simulink model "Flightinstrument"  (R2021b)
settings: Solver=VariableStepAuto  StartTime=0.0  StopTime=10.0  RelTol=1e-3
PreLoadFcn:
  | % Bus object: States
  | clear templateElems;
  | templateElems(1) = Simulink.BusElement;
  | templateElems(1).Name = 'V_body';
  | templateElems(1).Dimensions = [3 1];
  | templateElems(1).DimensionsMode = 'Fixed';
  | templateElems(1).DataType = 'double';
  | templateElems(1).SampleTime = -1;
  | templateElems(1).Complexity = 'real';
  | templateElems(1).SamplingMode = 'Sample based';
  | templateElems(1).Min = [];
  | templateElems(1).Max = [];
  | templateElems(1).DocUnits = '';
  | templateElems(1).Description = '';
  | 
  | templateElems(2) = Simulink.BusElement;
  | templateElems(2).Name = 'Omega_body';
  | templateElems(2).Dimensions = [3 1];
  | templateElems(2).DimensionsMode = 'Fixed';
  | templateElems(2).DataType = 'double';
  | templateElems(2).SampleTime = -1;
  | templateElems(2).Complexity = 'real';
  | templateElems(2).SamplingMode = 'Sample based';
  | templateElems(2).Min = [];
  | templateElems(2).Max = [];
  | templateElems(2).DocUnits = '';
  | templateElems(2).Description = '';
  | 
  | templateElems(3) = Simulink.BusElement;
  | templateElems(3).Name = 'Euler';
  | templateElems(3).Dimensions = [3 1];
  | templateElems(3).DimensionsMode = 'Fixed';
  | templateElems(3).DataType = 'double';
  | templateElems(3).SampleTime = -1;
  | templateElems(3).Complexity = 'real';
  | templateElems(3).SamplingMode = 'Sample based';
  | templateElems(3).Min = [];
  | templateElems(3).Max = [];
  | templateElems(3).DocUnits = '';
  | templateElems(3).Description = '';
  | 
  | templateElems(4) = Simulink.BusElement;
  | templateElems(4).Name = 'Accel_body';
  | templateElems(4).Dimensions = [3 1];
  | templateElems(4).DimensionsMode = 'Fixed';
  | templateElems(4).DataType = 'double';
  | templateElems(4).SampleTime = -1;
  | templateElems(4).Complexity = 'real';
  | templateElems(4).SamplingMode = 'Sample based';
  | templateElems(4).Min = [];
  | templateElems(4).Max = [];
  | templateElems(4).DocUnits = '';
  | templateElems(4).Description = '';
  | 
  | templateElems(5) = Simulink.BusElement;
  | templateElems(5).Name = 'dOmega_body';
  | templateElems(5).Dimensions = [3 1];
  | templateElems(5).DimensionsMode = 'Fixed';
  | templateElems(5).DataType = 'double';
  | templateElems(5).SampleTime = -1;
  | templateElems(5).Complexity = 'real';
  | templateElems(5).SamplingMode = 'Sample based';
  | templateElems(5).Min = [];
  | templateElems(5).Max = [];
  | templateElems(5).DocUnits = '';
  | templateElems(5).Description = '';
  | 
  | templateElems(6) = Simulink.BusElement;
  | templateElems(6).Name = 'V_ned';
  | templateElems(6).Dimensions = [3 1];
  | templateElems(6).DimensionsMode = 'Fixed';
  | templateElems(6).DataType = 'double';
  | templateElems(6).SampleTime = -1;
  | templateElems(6).Complexity = 'real';
  | templateElems(6).SamplingMode = 'Sample based';
  | templateElems(6).Min = [];
  | templateElems(6).Max = [];
  | templateElems(6).DocUnits = '';
  | templateElems(6).Description = '';
  | 
  | templateElems(7) = Simulink.BusElement;
  | templateElems(7).Name = 'X_ned';
  | templateElems(7).Dimensions = [3 1];
  | templateElems(7).DimensionsMode = 'Fixed';
  | templateElems(7).DataType = 'double';
  | templateElems(7).SampleTime = -1;
  | templateElems(7).Complexity = 'real';
  | templateElems(7).SamplingMode = 'Sample based';
  | templateElems(7).Min = [];
  | templateElems(7).Max = [];
  | templateElems(7).DocUnits = '';
  | templateElems(7).Description = '';
  | 
  | templateElems(8) = Simulink.BusElement;
  | templateElems(8).Name = 'LLA';
  | templateElems(8).Dimensions = [1 3];
  | templateElems(8).DimensionsMode = 'Fixed';
  | templateElems(8).DataType = 'double';
  | templateElems(8).SampleTime = -1;
  | templateElems(8).Complexity = 'real';
  | templateElems(8).SamplingMode = 'Sample based';
  | templateElems(8).Min = [];
  | templateElems(8).Max = [];
  | templateElems(8).DocUnits = '';
  | templateElems(8).Description = sprintf('Latitude, Longitude, Altitude');
  | 
  | templateElems(9) = Simulink.BusElement;
  | templateElems(9).Name = 'DCM_be';
  | templateElems(9).Dimensions = [3 3];
  | templateElems(9).DimensionsMode = 'Fixed';
  | templateElems(9).DataType = 'double';
  | templateElems(9).SampleTime = -1;
  | templateElems(9).Complexity = 'real';
  | templateElems(9).SamplingMode = 'Sample based';
  | templateElems(9).Min = [];
  | templateElems(9).Max = [];
  | templateElems(9).DocUnits = '';
  | templateElems(9).Description = '';
  | 
  | 
  | AirframeStatesBus = Simulink.Bus;
  | AirframeStatesBus.HeaderFile = '';
  | AirframeStatesBus.Description = '';
  | AirframeStatesBus.DataScope = 'Auto';
  | AirframeStatesBus.Alignment = -1;
  | AirframeStatesBus.Elements = templateElems;
  | clear templateElems;
undefined symbols (not defined in the file or in its folder): deg, Earth, ft, m, rad, s, WGS84
libraries: aerolibconvert2 x7, aerolibasang x3, shared6dof x1, aerolibadyn x1, aerolibactuator x1, aerolibtransform2 x1, aerolibnav x1
settings Model: Creator=asus  LastModifiedBy=asus
settings SolverCC: AlgebraicLoopSolver=TrustRegion  MinimalZcImpactIntegration=on
settings DebuggingCC: PregeneratedLibrarySubsystemCodeDiagnostic=none  SFMachineParentedDataDiag=warning  ArithmeticOperatorsInVariantConditions=warning
settings SFSimCC: SimUseLocalCustomCode=off
settings RTWCC: RTWUseLocalCustomCode=off

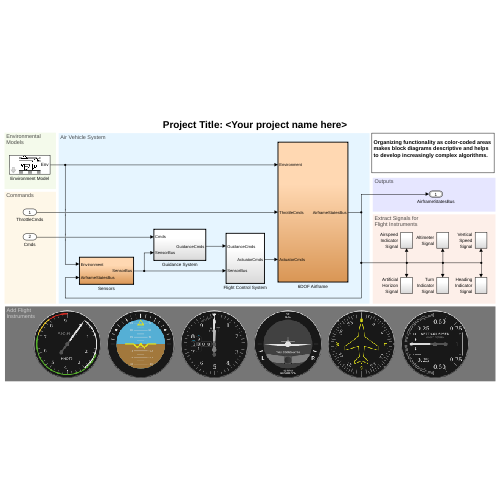
[thumbnail: Simulink's stored preview of the top-level diagram]
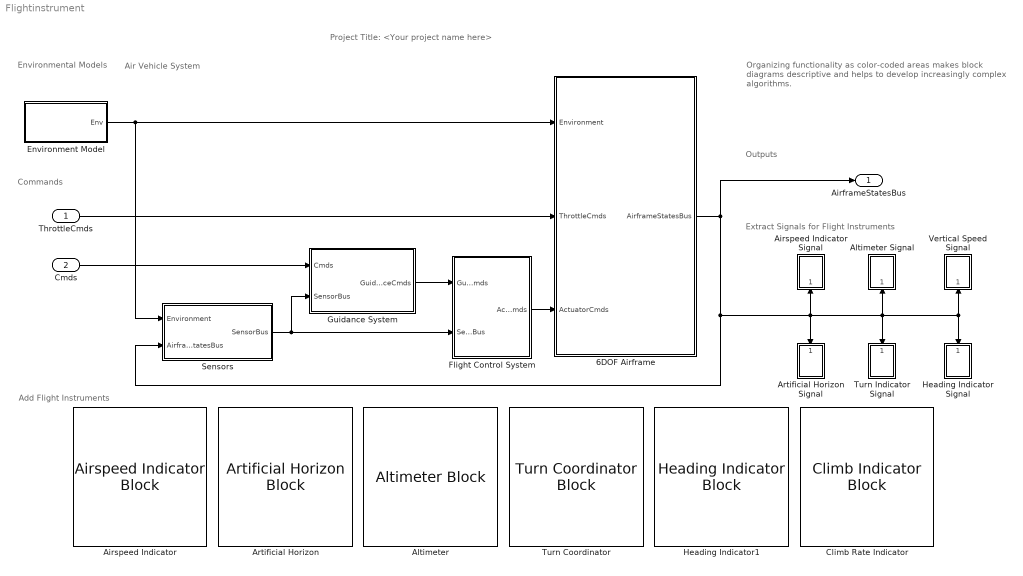
== system Flightinstrument ==
  note: Organizing functionality as color-coded areas makes block diagrams descriptive and helps to develop increasingly complex algorithms.
  note: Project Title: <Your project name here>
  note: Air Vehicle System
  note: Extract Signals for
      | Flight Instruments
  note: Add Flight
      | Instruments
  note: Outputs
  note: Environmental
      | Models
  note: Commands
  ThrottleCmds : Inport
  Cmds : Inport  Port=2
  6DOF Airframe : Subsystem  TreatAsAtomicUnit=on
  Airspeed Indicator Signal : Subsystem
  Airspeed Indicator : AirspeedIndicatorBlock  LabelPosition=Hide  ScaleMin=0  ScaleMax=9
  Altimeter : AltimeterBlock  LabelPosition=Hide
  Altimeter Signal : Subsystem
  Artificial Horizon Signal : Subsystem
  Artificial Horizon : ArtificialHorizonBlock  LabelPosition=Hide
  Climb Rate Indicator : ClimbIndicatorBlock  LabelPosition=Hide  ScaleMax=1000
  Environment Model : Subsystem  mask(Constant Environment Model){To=288, a=340, Po=101.3e3, AirDensity=1.229, ugvgwg=[0 0 0], pgqgrg=[0 0 0], g=[0 0 9.81]}
      mask prompts: To "Constant Temperature (K):"; a "Constant Speed of Sound (m/s):"; Po "Constant Pressure (Pa):"; AirDensity "Constant Air Density (kg/m^3):"; ugvgwg "Constant Wind Velocity [ug vg wg] (m/s):"; pgqgrg "Constant Wind Angular Rates [pg qg rg] (rad/s):"; g "Constant Gravitational Acceleration (m/s^2):"
      mask Help: helpview(fullfile(docroot,'toolbox','aeroblks','aeroblks.map'), 'environment1');
      mask TypeOptions To: Constant Atmosphere/To
      mask TypeOptions a: Constant Atmosphere/a
      mask TypeOptions Po: Constant Atmosphere/Po
      mask TypeOptions AirDensity: Constant Atmosphere/AirDensity
      mask TypeOptions ugvgwg: Constant Wind/ugvgwg
      mask TypeOptions pgqgrg: Constant Wind/pgqgrg
      mask TypeOptions g: Constant Gravity/g
      mask DialogControl Container4 Prompt: Atmospheric Model
      mask DialogControl Container6 Prompt: Wind Model
      mask DialogControl Container8 Prompt: Gravity Model
      mask Display:
      | image('aeroenvironment.bmp','center')
      | port_label('output',1,'Env')
  Flight Control System : Subsystem  TreatAsAtomicUnit=on
  Guidance System : Subsystem  TreatAsAtomicUnit=on
  Heading Indicator Signal : Subsystem
  Heading Indicator1 : HeadingIndicatorBlock  LabelPosition=Hide
  Sensors : Subsystem  TreatAsAtomicUnit=on  VariantControl=VSS_SENSORS_DYNAMICS
  Turn Indicator Signal : Subsystem
  Turn Coordinator : TurnCoordinatorBlock  LabelPosition=Hide
  Vertical Speed Signal : Subsystem
  AirframeStatesBus : Outport  OutDataTypeStr=Bus: AirframeStatesBus  VectorParamsAs1DForOutWhenUnconnected=off
  wires:
  6DOF Airframe/1(AirframeStatesBus) -> Sensors/2(AirframeStatesBus), Altimeter Signal/1(AirframeStatesBus), Heading Indicator Signal/1(AirframeStatesBus), Vertical Speed Signal/1(AirframeStatesBus), Turn Indicator Signal/1(AirframeStatesBus), Airspeed Indicator Signal/1(AirframeStatesBus), Artificial Horizon Signal/1(AirframeStatesBus), AirframeStatesBus/1
  Cmds/1 -> Guidance System/1(Cmds)
  Guidance System/1(GuidanceCmds) -> Flight Control System/1(GuidanceCmds)
  Sensors/1(SensorBus) -> Guidance System/2(SensorBus), Flight Control System/2(SensorBus)
  ThrottleCmds/1 -> 6DOF Airframe/2(ThrottleCmds)
  Environment Model/1(Env) -> Sensors/1(Environment), 6DOF Airframe/1(Environment)
  Flight Control System/1(ActuatorCmds) -> 6DOF Airframe/3(ActuatorCmds)

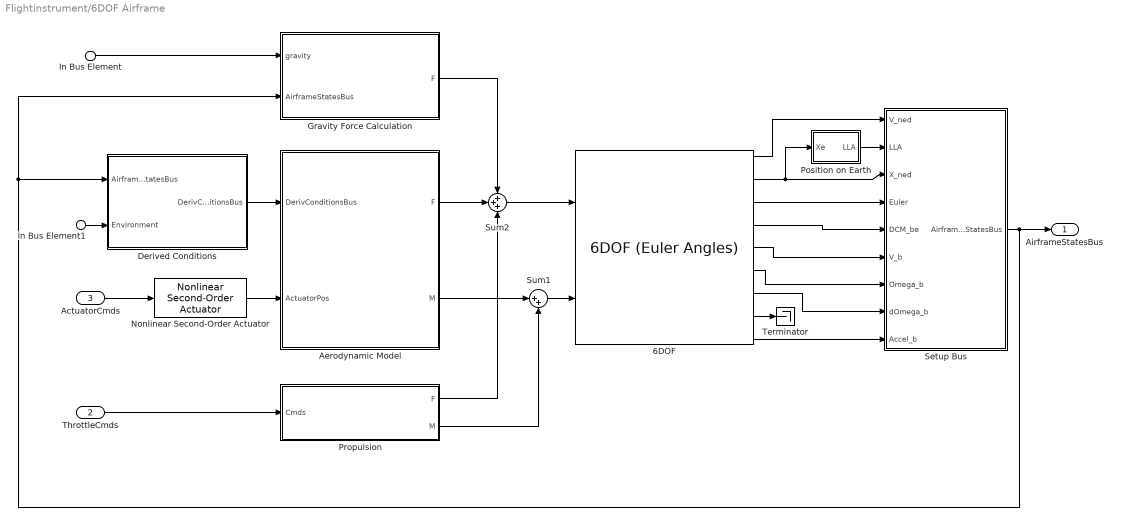
== system Flightinstrument/6DOF Airframe ==
  In Bus Element1 : Inport  PortName=Environment
  In Bus Element : Inport  PortName=Environment  Element=g
  ThrottleCmds : Inport  Port=2
  ActuatorCmds : Inport  Port=3
  6DOF : shared6dof/6DOF (Euler Angles)  units=Metric (MKS)  mtype=Fixed  rep=Euler Angles  xme_0=[0 0 -1000]  Vm_0=[100 0 0]  eul_0=[0 0 0]  pm_0=[0 0 0]  mass_0=1000  mass_e=0.5  mass_f=2.0  inertia=eye(3)  inertia_e=eye(3)  inertia_f=2*eye(3)  k_quat=Vehicle.SixDOF.quatGain  vre_flag=on  abi_flag=on  aMode=0  xme_statename=''  Vm_statename=''  eul_statename=''  quat_statename=''  pm_statename=''  mass_statename=''
      settings: SourceProductBaseCode=AE,PW,DR,MT,UV,VE
  Aerodynamic Model : Subsystem
  Derived Conditions : Subsystem
  Gravity Force Calculation : Subsystem
  Nonlinear Second-Order Actuator : aerolibactuator/Nonlinear Second-Order Actuator  wn_fin=1  z_fin=0.3  fin_max=20*pi/180  fin_min=-20*pi/180  fin_maxrate=500*pi/180  fin_act_0=0  fin_act_vel=0
      settings: SourceProductBaseCode=AE
  Position on Earth : Subsystem  Priority=1  TreatAsAtomicUnit=on
  Propulsion : Subsystem
  Setup Bus : Subsystem
  Sum1 : Sum  Inputs=|++  InputSameDT=on  SaturateOnIntegerOverflow=on  OutDataTypeStr=Inherit: Same as first input
  Sum2 : Sum  Inputs=+++  InputSameDT=on  SaturateOnIntegerOverflow=on  OutDataTypeStr=Inherit: Same as first input
  Terminator : Terminator
  AirframeStatesBus : Outport  OutDataTypeStr=Bus: AirframeStatesBus  VectorParamsAs1DForOutWhenUnconnected=off
  wires:
  Setup Bus/1(AirframeStatesBus) -> AirframeStatesBus/1, Gravity Force Calculation/2(AirframeStatesBus), Derived Conditions/1(AirframeStatesBus)
  6DOF/1 -> Setup Bus/1(V_ned)
  Derived Conditions/1(DerivConditionsBus) -> Aerodynamic Model/1(DerivConditionsBus)
  In Bus Element1/1 -> Derived Conditions/2(Environment)
  Aerodynamic Model/2(M) -> Sum1/1
  ThrottleCmds/1 -> Propulsion/1(Cmds)
  ActuatorCmds/1 -> Nonlinear Second-Order Actuator/1
  Nonlinear Second-Order Actuator/1 -> Aerodynamic Model/2(ActuatorPos)
  Propulsion/1(F) -> Sum2/3
  Propulsion/2(M) -> Sum1/2
  6DOF/5 -> Setup Bus/6(V_b)
  Aerodynamic Model/1(F) -> Sum2/2
  6DOF/4 -> Setup Bus/5(DCM_be)
  Gravity Force Calculation/1(F) -> Sum2/1
  In Bus Element/1 -> Gravity Force Calculation/1(gravity)
  6DOF/9 -> Setup Bus/9(Accel_b)
  Sum2/1 -> 6DOF/1
  Sum1/1 -> 6DOF/2
  6DOF/2 -> Position on Earth/1(Xe), Setup Bus/3(X_ned)
  6DOF/3 -> Setup Bus/4(Euler)
  6DOF/6 -> Setup Bus/7(Omega_b)
  6DOF/7 -> Setup Bus/8(dOmega_b)
  Position on Earth/1(LLA) -> Setup Bus/2(LLA)
  6DOF/8 -> Terminator/1

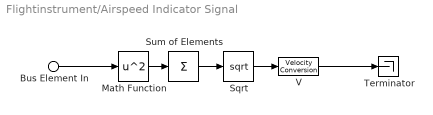
== system Flightinstrument/Airspeed Indicator Signal ==
  Bus Element In : Inport  PortName=AirframeStatesBus  Element=V_body
  Math Function : Math  Operator=square  SignedPower=on  SaturateOnIntegerOverflow=on
  Sqrt : Sqrt  SaturateOnIntegerOverflow=on
  Sum of Elements : Sum  Inputs=+
  Terminator : Terminator
  V : aerolibconvert2/Velocity Conversion  IU=m/s  OU=kts
  wires:
  Bus Element In/1 -> Math Function/1
  V/1 -> Terminator/1
  Sqrt/1 -> V/1
  Math Function/1 -> Sum of Elements/1
  Sum of Elements/1 -> Sqrt/1

== system Flightinstrument/Altimeter Signal ==
  Bus Element In : Inport  PortName=AirframeStatesBus  Element=LLA
  Altitude [ft] : aerolibconvert2/Length Conversion  IU=m  OU=ft
  Altitude [m] : Selector  InputPortWidth=3  IndexOptions=Index vector (dialog)  Indices=[3]  OutputSizes=1
  Terminator : Terminator
  wires:
  Bus Element In/1 -> Altitude [m]/1
  Altitude [ft]/1 -> Terminator/1
  Altitude [m]/1 -> Altitude [ft]/1

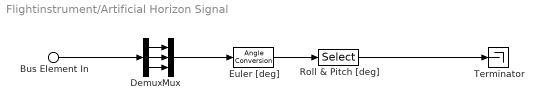
== system Flightinstrument/Artificial Horizon Signal ==
  Bus Element In : Inport  PortName=AirframeStatesBus  Element=Euler
  Demux : Demux  Outputs=3
  Euler [deg] : aerolibconvert2/Angle Conversion  IU=rad  OU=deg
  Mux : Mux  Inputs=3
  Roll & Pitch [deg] : Selector  InputPortWidth=3  IndexOptions=Index vector (dialog)  Indices=[1 2]  OutputSizes=1
  Terminator : Terminator
  wires:
  Roll & Pitch [deg]/1 -> Terminator/1
  Mux/1 -> Euler [deg]/1
  Demux/3 -> Mux/3
  Demux/1 -> Mux/1
  Demux/2 -> Mux/2
  Bus Element In/1 -> Demux/1
  Euler [deg]/1 -> Roll & Pitch [deg]/1

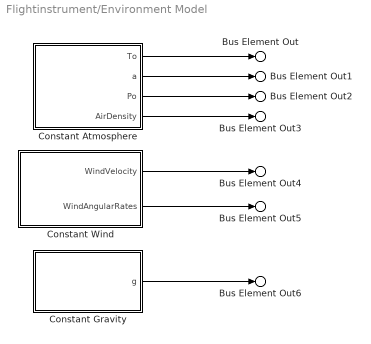
== system Flightinstrument/Environment Model ==
  Constant Atmosphere : Subsystem  VariantControl=atmosCONST  mask(Standard Atmospheric Constants){To=To, a=a, Po=Po, AirDensity=AirDensity}
      mask prompts: To "Constant Temperature (K):"; a "Constant Speed of Sound (m/s):"; Po "Constant Pressure (Pa):"; AirDensity "Constant Air Density (kg/m^3):"
  Constant Gravity : Subsystem  VariantControl=gravCONST  mask(Constant Gravitational Acceleration){g=g}
      mask prompts: g "Constant Gravitational Acceleration (m/s^2):"
  Constant Wind : Subsystem  VariantControl=windCONST  mask(Constant Wind Values){ugvgwg=ugvgwg, pgqgrg=pgqgrg}
      mask prompts: ugvgwg "Constant Wind Velocity (m/s):"; pgqgrg "Constant Wind Angular Rates (rad/s):"
  Bus Element Out : Outport  VectorParamsAs1DForOutWhenUnconnected=off  PortName=Env  Element=To
  Bus Element Out1 : Outport  VectorParamsAs1DForOutWhenUnconnected=off  PortName=Env  Element=a
  Bus Element Out2 : Outport  VectorParamsAs1DForOutWhenUnconnected=off  PortName=Env  Element=Po
  Bus Element Out3 : Outport  VectorParamsAs1DForOutWhenUnconnected=off  PortName=Env  Element=AirDensity
  Bus Element Out4 : Outport  VectorParamsAs1DForOutWhenUnconnected=off  PortName=Env  Element=WindVelocity
  Bus Element Out5 : Outport  VectorParamsAs1DForOutWhenUnconnected=off  PortName=Env  Element=WindAngularRates
  Bus Element Out6 : Outport  VectorParamsAs1DForOutWhenUnconnected=off  PortName=Env  Element=g
  wires:
  Constant Wind/2(WindAngularRates) -> Bus Element Out5/1
  Constant Atmosphere/3(Po) -> Bus Element Out2/1
  Constant Atmosphere/4(AirDensity) -> Bus Element Out3/1
  Constant Atmosphere/1(To) -> Bus Element Out/1
  Constant Wind/1(WindVelocity) -> Bus Element Out4/1
  Constant Atmosphere/2(a) -> Bus Element Out1/1
  Constant Gravity/1(g) -> Bus Element Out6/1

== system Flightinstrument/Flight Control System ==
  note: Add Flight Control System Algorithms
  GuidanceCmds : Inport
  SensorBus : Inport  Port=2
  Bus to Vector : BusToVector
  Terminator1 : Terminator
  ActuatorCmds : Outport  VectorParamsAs1DForOutWhenUnconnected=off
  wires:
  GuidanceCmds/1 -> Bus to Vector/1
  Bus to Vector/1 -> ActuatorCmds/1
  SensorBus/1 -> Terminator1/1

== system Flightinstrument/Guidance System ==
  note: Add Guidance System Algorithms
  Cmds : Inport
  SensorBus : Inport  Port=2
  Ground : Ground
  Terminator1 : Terminator
  Terminator2 : Terminator
  GuidanceCmds : Outport  VectorParamsAs1DForOutWhenUnconnected=off
  wires:
  Cmds/1 -> Terminator2/1
  Ground/1 -> GuidanceCmds/1
  SensorBus/1 -> Terminator1/1

== system Flightinstrument/Heading Indicator Signal ==
  note: Customize Deg from North per simulation
  Bus Element In : Inport  PortName=AirframeStatesBus  Element=Euler
  Deg from North : Bias
  Euler [deg] : aerolibconvert2/Angle Conversion  IU=rad  OU=deg
  Terminator : Terminator
  Yaw [deg] : Selector  InputPortWidth=3  IndexOptions=Index vector (dialog)  Indices=[3]  OutputSizes=1
  wires:
  Euler [deg]/1 -> Yaw [deg]/1
  Deg from North/1 -> Terminator/1
  Yaw [deg]/1 -> Deg from North/1
  Bus Element In/1 -> Euler [deg]/1

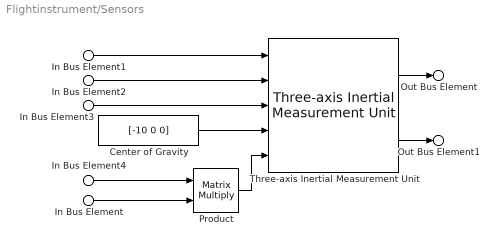
== system Flightinstrument/Sensors ==
  In Bus Element : Inport  PortName=Environment  Element=g
  In Bus Element1 : Inport  Port=2  PortName=AirframeStatesBus  Element=Accel_body
  In Bus Element2 : Inport  Port=2  PortName=AirframeStatesBus  Element=Omega_body
  In Bus Element3 : Inport  Port=2  PortName=AirframeStatesBus  Element=dOmega_body
  In Bus Element4 : Inport  Port=2  PortName=AirframeStatesBus  Element=DCM_be
  Center of Gravity : Constant  Value=[-10 0 0]
  Product : Product  Multiplication=Matrix(*)
  Three-axis Inertial Measurement Unit : aerolibnav/Three-axis Inertial Measurement Unit  units=Metric (MKS)  imu=[0 0 0]  i_Ts=0  dtype_a=on  w_a=190  z_a=0.707  a_sf_cc=[1 0 0; 0 1 0; 0 0 1]  a_bias=[0 0 0]  a_sat="[-inf  -inf  -inf  inf inf inf]"  dtype_g=on  w_g=190  z_g=0.707  g_sf_cc=[1 0 0; 0 1 0; 0 0 1]  g_bias=[0 0 0]  g_sens=[0 0 0]  g_sat="[-inf  -inf  -inf  inf inf inf]"  i_rand=on  i_seeds=[23093 23094 23095 23096 23097 23098]  i_pow=[0.001 0.001 0.001 0.0001 0.0001 0.0001]
  Out Bus Element : Outport  VectorParamsAs1DForOutWhenUnconnected=off  PortName=SensorBus  Element=Accel_body_meas
  Out Bus Element1 : Outport  VectorParamsAs1DForOutWhenUnconnected=off  PortName=SensorBus  Element=Omega_body_meas
  wires:
  In Bus Element/1 -> Product/2
  In Bus Element4/1 -> Product/1
  Three-axis Inertial Measurement Unit/2 -> Out Bus Element1/1
  Three-axis Inertial Measurement Unit/1 -> Out Bus Element/1
  Product/1 -> Three-axis Inertial Measurement Unit/5
  Center of Gravity/1 -> Three-axis Inertial Measurement Unit/4
  In Bus Element3/1 -> Three-axis Inertial Measurement Unit/3
  In Bus Element2/1 -> Three-axis Inertial Measurement Unit/2
  In Bus Element1/1 -> Three-axis Inertial Measurement Unit/1

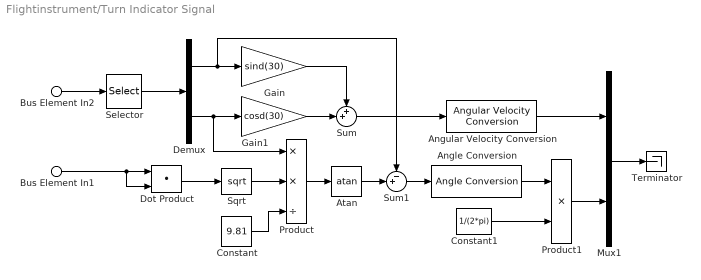
== system Flightinstrument/Turn Indicator Signal ==
  Bus Element In1 : Inport  PortName=AirframeStatesBus  Element=V_body
  Bus Element In2 : Inport  PortName=AirframeStatesBus  Element=Omega_body
  Angle Conversion : aerolibconvert2/Angle Conversion  IU=rad  OU=deg
  Angular Velocity Conversion : aerolibconvert2/Angular Velocity Conversion  IU=rad/s  OU=deg/s
  Atan : Trigonometry  Operator=atan
  Constant : Constant  Value=9.81
  Constant1 : Constant  Value=1/(2*pi)
  Demux : Demux  Outputs=2
  Dot Product : DotProduct  InputSameDT=on  OutDataTypeStr=Inherit: Inherit via internal rule
  Gain : Gain  Gain=sind(30)
  Gain1 : Gain  Gain=cosd(30)
  Mux1 : Mux  Inputs=2
  Product : Product  Inputs=**/
  Product1 : Product  Inputs=**
  Selector : Selector  InputPortWidth=3  IndexOptions=Index vector (dialog)  Indices=[1 3]  OutputSizes=1
  Sqrt : Sqrt  SaturateOnIntegerOverflow=on
  Sum : Sum  Inputs=++|
  Sum1 : Sum  Inputs=-+|
  Terminator : Terminator
  wires:
  Product1/1 -> Mux1/2
  Constant1/1 -> Product1/2
  Sum1/1 -> Angle Conversion/1
  Atan/1 -> Sum1/2
  Constant/1 -> Product/3
  Product/1 -> Atan/1
  Sqrt/1 -> Product/2
  Bus Element In1/1 -> Dot Product/1, Dot Product/2
  Dot Product/1 -> Sqrt/1
  Sum/1 -> Angular Velocity Conversion/1
  Gain1/1 -> Sum/2
  Gain/1 -> Sum/1
  Demux/2 -> Gain1/1, Product/1
  Demux/1 -> Sum1/1, Gain/1
  Selector/1 -> Demux/1
  Bus Element In2/1 -> Selector/1
  Angular Velocity Conversion/1 -> Mux1/1
  Angle Conversion/1 -> Product1/1
  Mux1/1 -> Terminator/1

== system Flightinstrument/Vertical Speed Signal ==
  Bus Element In : Inport  PortName=AirframeStatesBus  Element=V_ned
  Gain : Gain  Gain=-1/1000
  Terminator : Terminator
  Vd [ft/min] : aerolibconvert2/Velocity Conversion  IU=m/s  OU=ft/min
  Vd [m/s] : Selector  InputPortWidth=3  IndexOptions=Index vector (dialog)  Indices=[3]  OutputSizes=1
  wires:
  Gain/1 -> Terminator/1
  Bus Element In/1 -> Vd [m/s]/1
  Vd [m/s]/1 -> Vd [ft/min]/1
  Vd [ft/min]/1 -> Gain/1

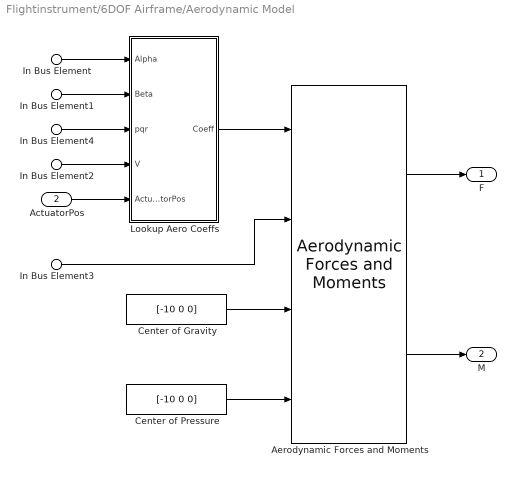
== system Flightinstrument/6DOF Airframe/Aerodynamic Model ==
  In Bus Element : Inport  PortName=DerivConditionsBus  Element=Alpha
  In Bus Element1 : Inport  PortName=DerivConditionsBus  Element=Beta
  In Bus Element2 : Inport  PortName=DerivConditionsBus  Element=Airspeed
  In Bus Element3 : Inport  PortName=DerivConditionsBus  Element=qbar
  In Bus Element4 : Inport  PortName=DerivConditionsBus  Element=Omega_total
  ActuatorPos : Inport  Port=2
  "Aerodynamic Forces and Moments " : aerolibadyn/Aerodynamic Forces and Moments   inputAxes=Body  outputForceAxes=Body  outputMomentAxes=Body  S=1  b=1  cbar=1
  Center of Gravity : Constant  Value=[-10 0 0]
  Center of Pressure : Constant  Value=[-10 0 0]
  Lookup Aero Coeffs : Subsystem
  F : Outport  Unit=N  VectorParamsAs1DForOutWhenUnconnected=off
  M : Outport  Port=2  Unit=N  VectorParamsAs1DForOutWhenUnconnected=off
  wires:
  In Bus Element4/1 -> Lookup Aero Coeffs/3(pqr)
  In Bus Element3/1 -> "Aerodynamic Forces and Moments "/2
  In Bus Element2/1 -> Lookup Aero Coeffs/4(V)
  In Bus Element1/1 -> Lookup Aero Coeffs/2(Beta)
  Center of Pressure/1 -> "Aerodynamic Forces and Moments "/4
  Center of Gravity/1 -> "Aerodynamic Forces and Moments "/3
  ActuatorPos/1 -> Lookup Aero Coeffs/5(ActuatorPos)
  Lookup Aero Coeffs/1(Coeff) -> "Aerodynamic Forces and Moments "/1
  "Aerodynamic Forces and Moments "/1 -> F/1
  "Aerodynamic Forces and Moments "/2 -> M/1
  In Bus Element/1 -> Lookup Aero Coeffs/1(Alpha)

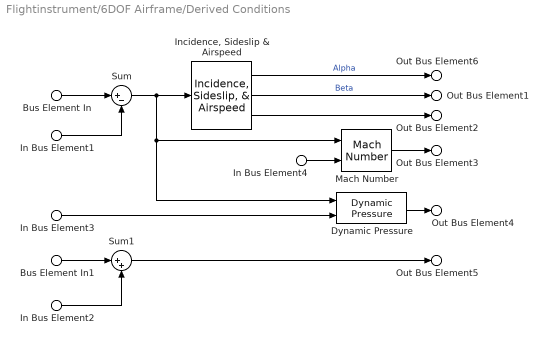
== system Flightinstrument/6DOF Airframe/Derived Conditions ==
  Bus Element In : Inport  PortName=AirframeStatesBus  Element=V_body
  Bus Element In1 : Inport  PortName=AirframeStatesBus  Element=Omega_body
  In Bus Element1 : Inport  Port=2  PortName=Environment  Element=WindVelocity
  In Bus Element2 : Inport  Port=2  PortName=Environment  Element=WindAngularRates
  In Bus Element3 : Inport  Port=2  PortName=Environment  Element=AirDensity
  In Bus Element4 : Inport  Port=2  PortName=Environment  Element=a
  Dynamic Pressure : aerolibasang/Dynamic Pressure
  "Incidence, Sideslip & Airspeed" : aerolibasang/Incidence, Sideslip, & Airspeed
  Mach Number : aerolibasang/Mach Number
      settings: SourceProductBaseCode=AE
  Sum : Sum  Inputs=|+-  InputSameDT=on  SaturateOnIntegerOverflow=on  OutDataTypeStr=Inherit: Same as first input
  Sum1 : Sum  Inputs=|++  InputSameDT=on  SaturateOnIntegerOverflow=on  OutDataTypeStr=Inherit: Same as first input
  Out Bus Element6 : Outport  VectorParamsAs1DForOutWhenUnconnected=off  PortName=DerivConditionsBus  Element=Alpha
  Out Bus Element1 : Outport  VectorParamsAs1DForOutWhenUnconnected=off  PortName=DerivConditionsBus  Element=Beta
  Out Bus Element2 : Outport  VectorParamsAs1DForOutWhenUnconnected=off  PortName=DerivConditionsBus  Element=Airspeed
  Out Bus Element3 : Outport  VectorParamsAs1DForOutWhenUnconnected=off  PortName=DerivConditionsBus  Element=Mach
  Out Bus Element4 : Outport  VectorParamsAs1DForOutWhenUnconnected=off  PortName=DerivConditionsBus  Element=qbar
  Out Bus Element5 : Outport  VectorParamsAs1DForOutWhenUnconnected=off  PortName=DerivConditionsBus  Element=Omega_total
  wires:
  In Bus Element1/1 -> Sum/2
  In Bus Element2/1 -> Sum1/2
  Sum1/1 -> Out Bus Element5/1
  Bus Element In1/1 -> Sum1/1
  "Incidence, Sideslip & Airspeed"/1 -> Out Bus Element6/1  "Alpha"
  "Incidence, Sideslip & Airspeed"/2 -> Out Bus Element1/1  "Beta"
  In Bus Element4/1 -> Mach Number/2
  Bus Element In/1 -> Sum/1
  Sum/1 -> "Incidence, Sideslip & Airspeed"/1, Mach Number/1, Dynamic Pressure/1
  Mach Number/1 -> Out Bus Element3/1
  In Bus Element3/1 -> Dynamic Pressure/2
  Dynamic Pressure/1 -> Out Bus Element4/1
  "Incidence, Sideslip & Airspeed"/3 -> Out Bus Element2/1

== system Flightinstrument/6DOF Airframe/Gravity Force Calculation ==
  gravity : Inport  Unit=m/s^2
  Bus Element In : Inport  Port=2  PortName=AirframeStatesBus  Element=DCM_be
  Airframe Mass : Gain  Gain=1000
  Product : Product  Multiplication=Matrix(*)
  F : Outport  Unit=N  VectorParamsAs1DForOutWhenUnconnected=off
  wires:
  gravity/1 -> Airframe Mass/1
  Airframe Mass/1 -> Product/2  "gravity force NED"
  Product/1 -> F/1
  Bus Element In/1 -> Product/1

== system Flightinstrument/6DOF Airframe/Position on Earth ==
  Xe : Inport  Unit=m
  Flat Earth to LLA : aerolibtransform2/Flat Earth to LLA  units=Metric (MKS)  ptype=Earth (WGS84)  F=1/298.257223563  R=6378137  refPosPort=off  LL0=[0 10]  psi=0
  Mux : Mux  Inputs=2
  href : Constant  Value=0
  LLA : Outport  VectorParamsAs1DForOutWhenUnconnected=off
  wires:
  Mux/1 -> LLA/1
  Xe/1 -> Flat Earth to LLA/1
  Flat Earth to LLA/1 -> Mux/1
  Flat Earth to LLA/2 -> Mux/2
  href/1 -> Flat Earth to LLA/2

== system Flightinstrument/6DOF Airframe/Propulsion ==
  note: Add lookup tables or dynamics for propulsion
  Cmds : Inport
  "Fx, Fy, Fz" : Constant  Value=[0 0 0]
  "Mx, My, Mz" : Constant  Value=[0 0 0]
  Terminator : Terminator
  F : Outport  Unit=N  VectorParamsAs1DForOutWhenUnconnected=off
  M : Outport  Port=2  Unit=N*m  VectorParamsAs1DForOutWhenUnconnected=off
  wires:
  "Mx, My, Mz"/1 -> M/1
  "Fx, Fy, Fz"/1 -> F/1
  Cmds/1 -> Terminator/1

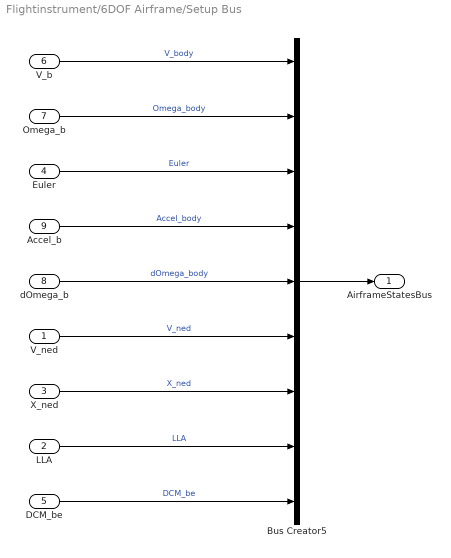
== system Flightinstrument/6DOF Airframe/Setup Bus ==
  V_ned : Inport  PortDimensions=3
  LLA : Inport  Port=2  PortDimensions=3
  X_ned : Inport  Port=3  PortDimensions=3
  Euler : Inport  Port=4  PortDimensions=3
  DCM_be : Inport  Port=5  PortDimensions=[3 3]
  V_b : Inport  Port=6  PortDimensions=3
  Omega_b : Inport  Port=7  PortDimensions=3
  dOmega_b : Inport  Port=8  PortDimensions=3
  Accel_b : Inport  Port=9  PortDimensions=3
  Bus Creator5 : BusCreator  Inputs=9  OutDataTypeStr=Bus: AirframeStatesBus
  AirframeStatesBus : Outport  OutDataTypeStr=Bus: AirframeStatesBus  VectorParamsAs1DForOutWhenUnconnected=off
  wires:
  Bus Creator5/1 -> AirframeStatesBus/1
  V_b/1 -> Bus Creator5/1  "V_body"
  Omega_b/1 -> Bus Creator5/2  "Omega_body"
  Euler/1 -> Bus Creator5/3  "Euler"
  X_ned/1 -> Bus Creator5/7  "X_ned"
  Accel_b/1 -> Bus Creator5/4  "Accel_body"
  LLA/1 -> Bus Creator5/8  "LLA"
  dOmega_b/1 -> Bus Creator5/5  "dOmega_body"
  DCM_be/1 -> Bus Creator5/9  "DCM_be"
  V_ned/1 -> Bus Creator5/6  "V_ned"

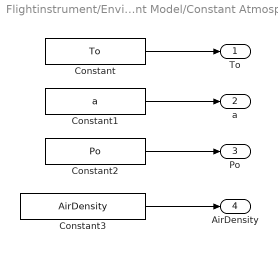
== system Flightinstrument/Environment Model/Constant Atmosphere ==
  Constant : Constant  Value=To
  Constant1 : Constant  Value=a
  Constant2 : Constant  Value=Po
  Constant3 : Constant  Value=AirDensity
  To : Outport  VectorParamsAs1DForOutWhenUnconnected=off
  a : Outport  Port=2  VectorParamsAs1DForOutWhenUnconnected=off
  Po : Outport  Port=3  VectorParamsAs1DForOutWhenUnconnected=off
  AirDensity : Outport  Port=4  VectorParamsAs1DForOutWhenUnconnected=off
  wires:
  Constant1/1 -> a/1
  Constant/1 -> To/1
  Constant2/1 -> Po/1
  Constant3/1 -> AirDensity/1

== system Flightinstrument/Environment Model/Constant Gravity ==
  Standard Gravity : Constant  Value=g
  g : Outport  VectorParamsAs1DForOutWhenUnconnected=off
  wires:
  Standard Gravity/1 -> g/1

== system Flightinstrument/Environment Model/Constant Wind ==
  Reshape : Reshape  OutputDimensionality=Column vector (2-D)
  Reshape1 : Reshape  OutputDimensionality=Column vector (2-D)
  pg,qg,rg : Constant  Value=pgqgrg
  ug,vg,wg : Constant  Value=ugvgwg
  WindVelocity : Outport  VectorParamsAs1DForOutWhenUnconnected=off
  WindAngularRates : Outport  Port=2  VectorParamsAs1DForOutWhenUnconnected=off
  wires:
  pg,qg,rg/1 -> Reshape1/1
  ug,vg,wg/1 -> Reshape/1
  Reshape/1 -> WindVelocity/1
  Reshape1/1 -> WindAngularRates/1

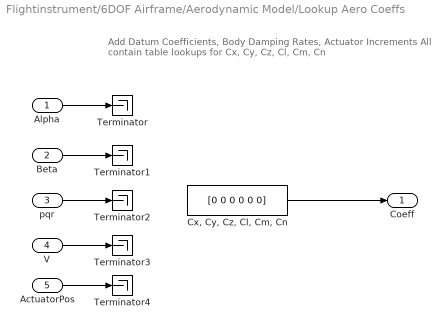
== system Flightinstrument/6DOF Airframe/Aerodynamic Model/Lookup Aero Coeffs ==
  note: Add Datum Coefficients, Body Damping Rates, Actuator Increments
      | All contain table lookups for Cx, Cy, Cz, Cl, Cm, Cn
  Alpha : Inport  Unit=rad
  Beta : Inport  Port=2  Unit=rad
  pqr : Inport  Port=3  Unit=rad
  V : Inport  Port=4  Unit=rad
  ActuatorPos : Inport  Port=5  Unit=rad
  "Cx, Cy, Cz, Cl, Cm, Cn" : Constant  Value=[0 0 0 0 0 0]
  Terminator{,1..4} (5 alike) : Terminator
  Coeff : Outport  VectorParamsAs1DForOutWhenUnconnected=off
  wires:
  "Cx, Cy, Cz, Cl, Cm, Cn"/1 -> Coeff/1
  Beta/1 -> Terminator1/1
  pqr/1 -> Terminator2/1
  V/1 -> Terminator3/1
  ActuatorPos/1 -> Terminator4/1
  Alpha/1 -> Terminator/1
